simulink model "BD_SER2"  (Simulink 4.1.1)
settings: Solver=ode1  SolverMode=SingleTasking  StartTime=0.0  StopTime=max(cyc_mph(:,1))  FixedStep=1  MaxStep=1  RelTol=1e-3  AbsTol=1e-3
undefined symbols (not defined in the file): air_cp, amb_tmp, cyc_avg_time, cyc_cargo_mass, cyc_elevation_init, cyc_filter_bool, cyc_grade, cyc_mph, enable_stop, ess_cap_scale, ess_coulombic_eff, ess_init_soc, ess_max_ah_cap, ess_max_volts, ess_min_volts, ess_mod_airflow, ess_mod_cp, ess_mod_init_tmp, ess_module_mass, ess_module_num, ess_on, ess_res_scale_coef, ess_res_scale_fun, ess_set_tmp, ess_th_calc, ess_th_res_off, ess_th_res_on, ess_tmp, ess_voc, ex_calc, fc_ct_trq, fc_emis, fc_inertia, fc_map_spd, fc_max_trq, fc_spd_scale, fc_trq_scale, fd_inertia, fd_loss, fd_ratio, gb_dnshift_load, gb_dnshift_spd, gb_gears_num, gb_inertia, gb_num_init, gb_ratio, gb_shift_delay, gb_spd_scale, gb_trq_scale, gb_upshift_load, gb_upshift_spd, gc_inertia, gc_map_spd, gc_map_trq, gc_max_crrnt, gc_max_trq, gc_outpwr_map, gc_overtrq_factor, gc_spd_scale, gc_trq_scale ... (+37)
libraries: lib_wheel2 x12, lib_accessory2 x4, lib_controls2 x3, lib_etc x2, lib_help x2, lib_fuel_converter x2, lib_drive_cycle2 x1, lib_interactive x1, lib_drive_cycle x1, lib_exhaust x1, lib_fuel_converter3 x1
(part 1 of 15)
settings Model: ExecutionOrder=on  LastModifiedBy=mokeefe  ModifiedComment=mokeefe -- Thu Apr 17 14:19:28 2003 -- Version 1.44  SaveTime=off  SaveOutput=off  LimitDataPoints=off  UnconnectedLineMsg=none  RTWOptions="-aEnforceIntegerDowncast=1 -aExtMode=0 -aFoldNonRolledExpr=1 -aForceParamTrailComments=0 -aGenerateComments=1 -aIgnoreCustomStorageClasses=1 -aIncHierarchyInIds=0 -aInlineInvariantSignals=1 -aInlineParameters=0 -aLocalBlockOutputs=1 -aLogVarNameModifier=\"rt_\" -aRTWVerbose=1 -aRollThreshold=5 -aShowEliminatedStatements=1"  RTWTemplateMakefile=grt_vc.tmf  ExtModeTrigMode=oneshot  ExtModeArmWhenConnect=off
settings Model: ModifiedHistory=|
  | mokeefe -- Thu Apr 17 14:19:28 2003 -- Version 1.44
  | 
  | 
  | abrooker -- Tue May 14 11:48:19 2002 -- Version 1.43
  | 
  | 
  | mokeefe -- Thu Apr 18 08:06:50 2002 -- Version 1.42
  | saving the model:
  | o "without the model browser open"
  | o with only top-level screen visible
  | o and with "fit to view" enabled

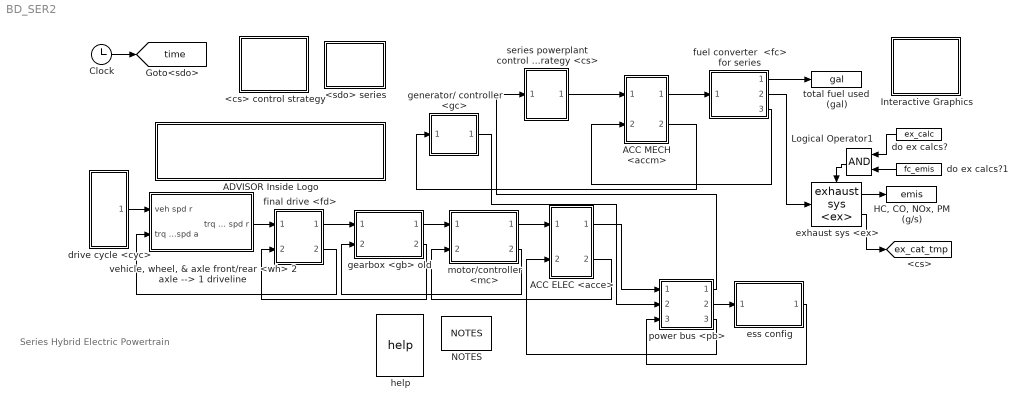
== system BD_SER2 ==
  note: Series Hybrid Electric
      | Powertrain
  <cs> control strategy : Subsystem
      settings: RTWFcnNameOpts=Auto  RTWFileNameOpts=Auto
      mask Display: image(imread('bdi_cs.jpg'))
  <sdo> series : Subsystem
      settings: RTWFcnNameOpts=Auto  RTWFileNameOpts=Auto
      mask Display: image(imread('bdi_sdo.jpg'))
  ACC ELEC <acce> : Subsystem  AncestorBlock=lib_accessory2/ACC ELEC <acce>  mask(Stand-Alone Electrical Accessory Mask){generalName='acce', logPick=Log, initFileName={}, modCell={}, imgFileName='bdi_acc_elec.bmp', DEBUG=OFF}
      mask prompts: generalName "General Name of this Component [char]"; logPick "Log Variables to Workspace?"; initFileName "Initialization File(s) [cell array of char]"; modCell "Modification Cell [2 column cell array of param and val]"; imgFileName "Icon image file name [char--evaluated]"
      mask init:
      | % initialization via m-file script
      | advSACompMaskInit;
      settings: RTWFcnNameOpts=Auto  RTWFileNameOpts=Auto
      mask StyleString: edit,popup(Don't Log|Log),edit,edit,edit,popup(ON|OFF)
      mask Display: image(imread(imgFileName))
  ACC MECH <accm> : Subsystem  AncestorBlock=lib_accessory2/ACC MECH <accm>  mask(Stand-Alone Mechanical Accessory Mask){generalName='accm', logPick=Log, initFileName={}, modCell={}, imgFileName='bdi_acc_pic.bmp', DEBUG=OFF}
      mask prompts: generalName "General Name of this Component [char]"; logPick "Log Variables to Workspace?"; initFileName "Initialization File(s) [cell array of char]"; modCell "Modification Cell [2 column cell array of param and val]"; imgFileName "Icon image file name [char--evaluated]"
      mask init:
      | % initialization via m-file script
      | advSACompMaskInit;
      settings: RTWFcnNameOpts=Auto  RTWFileNameOpts=Auto
      mask StyleString: edit,popup(Don't Log|Log),edit,edit,edit,popup(ON|OFF)
      mask Display: image(imread(imgFileName))
  ADVISOR Inside Logo : Subsystem
      settings: RTWFcnNameOpts=Auto  RTWFileNameOpts=Auto
      mask Display: image(imread('advisorInside.jpg'))
  Clock : Clock
      settings: DisplayTime=off  Decimation=10
  "HC, CO, NOx, PM (g/s)" : ToWorkspace  VariableName=emis  SampleTime=0  SaveFormat=Array
  Interactive Graphics : Subsystem  BlockChoice=off
      settings: AttributesFormatString=%<BlockChoice>  TemplateBlock=lib_interactive/Interactive Graphics  MemberBlocks=off,on  RTWFcnNameOpts=Auto  RTWFileNameOpts=Auto
  Logical Operator1 : Logic  Orientation=left  Operator=AND  Inputs=2
  NOTES : lib_help/NOTES
  do ex calcs? : Constant  Orientation=left  Value=ex_calc
  do ex calcs?1 : Constant  Orientation=left  Value=fc_emis
  drive cycle <cyc> : Subsystem  AncestorBlock=lib_drive_cycle2/drive cycle <cyc>  mask(Stand-Alone Drive Cycle Mask){generalName='cyc', logPick=Log, initFileName={}, modCell={}, imgFileName='bdi_cyc.jpg', DEBUG=OFF, veh_mass=veh_mass}
      mask prompts: generalName "General Name of this Component [char]"; logPick "Log Variables to Workspace?"; initFileName "Initialization File(s) [cell array of char]"; modCell "Modification Cell [2 column cell array of param and val]"; imgFileName "Icon image file name [char--evaluated]"; veh_mass "Vehicle Mass (kg)"
      mask init:
      | % initialization via m-file script
      | advSACompMaskInit;
      settings: RTWFcnNameOpts=Auto  RTWFileNameOpts=Auto
      mask StyleString: edit,popup(Don't Log|Log),edit,edit,edit,popup(ON|OFF),edit
      mask Display: image(imread(imgFileName))
  ess config : Subsystem  BlockChoice=energy storage <ess>
      link override energy storage <ess>/controlTag: GotoTag=essControl
      link override energy storage <ess>/energy storage <ess>/Model/compute current/enhancedToWorkspace2/To Workspace: VariableName=ess_current  SampleTime=-1  SaveFormat=Array
      link override energy storage <ess>/energy storage <ess>/Model/enhancedToWorkspace/To Workspace: VariableName=ess_pwr_out_r  SampleTime=-1  SaveFormat=Array
      link override energy storage <ess>/energy storage <ess>/Model/enhancedToWorkspace1/To Workspace: VariableName=ess_pwr_loss_a  SampleTime=-1  SaveFormat=Array
      link override energy storage <ess>/energy storage <ess>/Model/enhancedToWorkspace2/To Workspace: VariableName=ess_mod_tmp  SampleTime=-1  SaveFormat=Array
      link override energy storage <ess>/energy storage <ess>/Model/enhancedToWorkspace3/To Workspace: VariableName=ess_air_tmp  SampleTime=-1  SaveFormat=Array
      link override energy storage <ess>/energy storage <ess>/Model/enhancedToWorkspace4/To Workspace: VariableName=ess_air_th_pwr  SampleTime=-1  SaveFormat=Array
      link override energy storage <ess>/energy storage <ess>/Model/enhancedToWorkspace5/To Workspace: VariableName=ess_pwr_out_a  SampleTime=-1  SaveFormat=Array
      link override energy storage <ess>/reqOutTag: GotoTag=essReqOut  TagVisibility=global
      link override energy storage <ess>/sensorsTag: GotoTag=essSensors  TagVisibility=global
      settings: AttributesFormatString=%<BlockChoice>  TemplateBlock=lib_energy_storage2/ess config  MemberBlocks="Ultracapacitor  System,energy storage <ess>,energy storage <ess> RC,energy storage <ess> nnet,energy storage <ess> Saber,energy storage <ess> fundamental model,energy storage <ess> optima fundamental model"  RTWFcnNameOpts=Auto  RTWFileNameOpts=Auto
  exhaust sys <ex> : lib_exhaust/exhaust sys <ex>
  final drive <fd> : Subsystem  AncestorBlock=lib_transmission2/final drive <fd>  mask(Stand-Alone Final Drive Mask){generalName='fd', logPick=Log, initFileName={}, modCell={}, imgFileName='bdi_fd.jpg', DEBUG=OFF}
      mask prompts: generalName "General Name of this Component [char]"; logPick "Log Variables to Workspace?"; initFileName "Initialization File(s) [cell array of char]"; modCell "Modification Cell [2 column cell array of param and val]"; imgFileName "Icon image file name [char--evaluated]"
      mask init:
      | % initialization via m-file script
      | advSACompMaskInit;
      settings: RTWFcnNameOpts=Auto  RTWFileNameOpts=Auto
      mask StyleString: edit,popup(Don't Log|Log),edit,edit,edit,popup(ON|OFF)
      mask Display: image(imread(imgFileName))
  fuel converter  <fc> for series : Subsystem  AncestorBlock=|  mask(Stand-Alone IC ENGINE Mask (Series Hybrid)){generalName='fc', logPick=Log, initFileName={}, modCell={}, imgFileName='bdi_fc.jpg', DEBUG=OFF}
      | lib_fuel_converter3/fuel
      | converter
      |  <fc> for series
      mask prompts: generalName "General Name of this Component [char]"; logPick "Log Variables to Workspace?"; initFileName "Initialization File(s) [cell array of char]"; modCell "Modification Cell [2 column cell array of param and val]"; imgFileName "Icon image file name [char--evaluated]"
      mask init:
      | % initialization via m-file script
      | advSACompMaskInit;
      settings: RTWFcnNameOpts=Auto  RTWFileNameOpts=Auto
      mask StyleString: edit,popup(Don't Log|Log),edit,edit,edit,popup(ON|OFF)
      mask Display: image(imread(imgFileName))
  gearbox <gb> old : Subsystem  AncestorBlock=lib_transmission2/gearbox <gb> old  mask(Stand-Alone Gearbox Mask){generalName='gb', logPick=Log, initFileName={}, modCell={}, imgFileName='bdi_gb.jpg', DEBUG=OFF}
      mask prompts: generalName "General Name of this Component [char]"; logPick "Log Variables to Workspace?"; initFileName "Initialization File(s) [cell array of char]"; modCell "Modification Cell [2 column cell array of param and val]"; imgFileName "Icon image file name [char--evaluated]"
      mask init:
      | % initialization via m-file script
      | advSACompMaskInit;
      settings: RTWFcnNameOpts=Auto  RTWFileNameOpts=Auto
      mask StyleString: edit,popup(Don't Log|Log),edit,edit,edit,popup(ON|OFF)
      mask Display: image(imread(imgFileName))
  generator/ controller <gc> : Subsystem  AncestorBlock=lib_electric_machine2/generator// controller <gc>  mask(Stand-Alone Generator/Controller Mask){generalName='gc', logPick=Log, initFileName={}, modCell={}, imgFileName='bdi_mc.jpg', DEBUG=OFF}
      mask prompts: generalName "General Name of this Component [char]"; logPick "Log Variables to Workspace?"; initFileName "Initialization File(s) [cell array of char]"; modCell "Modification Cell [2 column cell array of param and val]"; imgFileName "Icon image file name [char--evaluated]"
      mask init:
      | % initialization via m-file script
      | advSACompMaskInit;
      settings: RTWFcnNameOpts=Auto  RTWFileNameOpts=Auto
      mask StyleString: edit,popup(Don't Log|Log),edit,edit,edit,popup(ON|OFF)
      mask Display: image(imread(imgFileName))
  help : lib_help/help
  motor/controller <mc> : Subsystem  AncestorBlock=lib_electric_machine2/motor//controller <mc>  mask(Stand-Alone Motor/Controller Mask){generalName='mc', logPick=Log, initFileName={}, modCell={}, imgFileName='bdi_mc.jpg', DEBUG=OFF}
      mask prompts: generalName "General Name of this Component [char]"; logPick "Log Variables to Workspace?"; initFileName "Initialization File(s) [cell array of char]"; modCell "Modification Cell [2 column cell array of param and val]"; imgFileName "Icon image file name [char--evaluated]"
      mask init:
      | % initialization via m-file script
      | advSACompMaskInit;
      settings: RTWFcnNameOpts=Auto  RTWFileNameOpts=Auto
      mask StyleString: edit,popup(Don't Log|Log),edit,edit,edit,popup(ON|OFF)
      mask Display: image(imread(imgFileName))
  power bus <pb> : Subsystem  AncestorBlock=lib_power_bus2/power bus <pb>  mask(Stand-Alone Power Bus Mask){generalName='pb', logPick=Log, initFileName={}, modCell={}, imgFileName='bdi_pb.jpg', DEBUG=OFF}
      mask prompts: generalName "General Name of this Component [char]"; logPick "Log Variables to Workspace?"; initFileName "Initialization File(s) [cell array of char]"; modCell "Modification Cell [2 column cell array of param and val]"; imgFileName "Icon image file name [char--evaluated]"
      mask init:
      | % initialization via m-file script
      | advSACompMaskInit;
      settings: RTWFcnNameOpts=Auto  RTWFileNameOpts=Auto
      mask StyleString: edit,popup(Don't Log|Log),edit,edit,edit,popup(ON|OFF)
      mask Display: image(imread(imgFileName))
  series powerplant control strategy <cs> : Subsystem  AncestorBlock=lib_controls2/series powerplant control strategy <cs>  mask(Stand-Alone Series Powerplant Control Strategy Mask){generalName='cs', logPick=Log, initFileName={}, modCell={}, imgFileName='bdi_hybrid_cntrl.jpg', DEBUG=OFF}
      mask prompts: generalName "General Name of this Component [char]"; logPick "Log Variables to Workspace?"; initFileName "Initialization File(s) [cell array of char]"; modCell "Modification Cell [2 column cell array of param and val]"; imgFileName "Icon image file name [char--evaluated]"
      mask init:
      | % initialization via m-file script
      | advSACompMaskInit;
      settings: RTWFcnNameOpts=Auto  RTWFileNameOpts=Auto
      mask StyleString: edit,popup(Don't Log|Log),edit,edit,edit,popup(ON|OFF)
      mask Display: image(imread(imgFileName))
  total fuel used  (gal) : ToWorkspace  VariableName=gal  SampleTime=0  SaveFormat=Array
  "vehicle, wheel, & axle front/rear <wh> 2 axle --> 1 driveline" : Subsystem  AncestorBlock=|  mask(Stand-Alone Vehicle, Wheel, & Axle Mask){generalName='veh', generalName01='wh', logPick=Log, initFileName={}, modCell={}, imgFileName='bdi_wh&veh.jpg', DEBUG=OFF}
      | lib_wheel2/vehicle, wheel, & axle
      | front//rear <wh>
      | 2 axle --> 1 driveline
      mask prompts: generalName "General Name of Vehicle Component [char]"; generalName01 "General Name of Wheel Component [char]"; logPick "Log Variables to Workspace?"; initFileName "Initialization File(s) for VEH and WH [cell array of char]"; modCell "Modification Cell [2 column cell array of param and val]"; imgFileName "Icon image file name [char--evaluated]"
      mask init:
      | % initialization via m-file script
      | advSACompMaskInit;
      settings: RTWFcnNameOpts=Auto  RTWFileNameOpts=Auto
      mask StyleString: edit,edit,popup(Don't Log|Log),edit,edit,edit,popup(ON|OFF)
      mask Display: image(imread(imgFileName))
  tag scope: ex_cat_tmp=global, time=global
  wires:
  gearbox <gb> old/1("torque and speed req'd at input side of gearbox (Nm), (rad/s)") -> motor/controller <mc>/1(trq and spd out requested)
  final drive <fd>/2("torque and speed avail. at output side of final drive (Nm), (rad/s)") -> "vehicle, wheel, & axle front/rear <wh> 2 axle --> 1 driveline"/2(trq & spd a)
  "vehicle, wheel, & axle front/rear <wh> 2 axle --> 1 driveline"/1(trq & spd r) -> final drive <fd>/1("torque and speed req'd at output side of final drive (Nm), (rad/s)")
  gearbox <gb> old/2("torque and speed avail. at output side of gearbox (Nm), (rad/s)") -> final drive <fd>/2("torque and speed avail. at input side of final drive (Nm), (rad/s)")
  final drive <fd>/1("torque and speed req'd at input side of final drive (Nm), (rad/s)") -> gearbox <gb> old/1("torque and speed req'd at output side of gearbox (Nm), (rad/s)")
  drive cycle <cyc>/1(req'd vehicle speed (m/s)) -> "vehicle, wheel, & axle front/rear <wh> 2 axle --> 1 driveline"/1(veh spd r)
  Clock/1 -> [time]
  fuel converter  <fc> for series/2(EO emis info) -> exhaust sys <ex>/1
  fuel converter  <fc> for series/1(fuel use) -> total fuel used  (gal)/1
  Logical Operator1/1 -> exhaust sys <ex>/Enable
  do ex calcs?/1 -> Logical Operator1/1
  exhaust sys <ex>/1 -> "HC, CO, NOx, PM (g/s)"/1
  do ex calcs?1/1 -> Logical Operator1/2
  generator/ controller <gc>/1(generator output power (W)) -> power bus <pb>/2(power available from source one (W))
  ess config/1(power available to bus (W)) -> power bus <pb>/3(power available from source two (W))
  power bus <pb>/2(power req'd from source two (W)) -> ess config/1(power req'd into bus (W))
  motor/controller <mc>/2("trq and spd out achieved ") -> gearbox <gb> old/2("torque and speed avail. at input side of gearbox (Nm), (rad/s)")
  power bus <pb>/1(power req'd from source one (W)) -> series powerplant control strategy <cs>/1(power req'd by bus (W))
  exhaust sys <ex>/2 -> [ex_cat_tmp]
  series powerplant control strategy <cs>/1("engine torque and speed (Nm), (rad/s)") -> ACC MECH <accm>/1(trq and spd out requested)
  ACC MECH <accm>/1(trq and spd in  requested) -> fuel converter  <fc> for series/1(torque and speed  req'd at engine  output shaft (Nm))
  fuel converter  <fc> for series/3("torque and speed  avail. to driveline (Nm), (rad/s)") -> ACC MECH <accm>/2(trq and spd in achieved)
  ACC MECH <accm>/2("trq and spd out achieved ") -> generator/ controller <gc>/1("torque and speed supplied to rotor (Nm), (rad/s)")
  motor/controller <mc>/1(electric power in  requested) -> ACC ELEC <acce>/1(elec pwr out r (W))
  ACC ELEC <acce>/1(elec pwr in r (W)) -> power bus <pb>/1(req'd power output (W))
  power bus <pb>/3(output power  available at bus) -> ACC ELEC <acce>/2(elec pwr in a (W))
  ACC ELEC <acce>/2(elec pwr out a (W)) -> motor/controller <mc>/2(electric power in achieved)

== system BD_SER2/<cs> control strategy ==
  Drive Cycle : Subsystem
      settings: RTWFcnNameOpts=Auto  RTWFileNameOpts=Auto
  Electrical Accessories : Subsystem
      settings: RTWFcnNameOpts=Auto  RTWFileNameOpts=Auto
  Gearbox Control manual shift logic for series : Subsystem
      settings: RTWFcnNameOpts=Auto  RTWFileNameOpts=Auto
  Generator : Subsystem
      settings: RTWFcnNameOpts=Auto  RTWFileNameOpts=Auto
  Hybrid Control Strategy : Subsystem
      settings: RTWFcnNameOpts=Auto  RTWFileNameOpts=Auto
      mask Display: image(imread('bdi_hybrid_cntrl.jpg'))
  IC Engine Control Series Hybrid : Subsystem
      settings: RTWFcnNameOpts=Auto  RTWFileNameOpts=Auto
  Mechanical Accessories : Subsystem
      settings: RTWFcnNameOpts=Auto  RTWFileNameOpts=Auto
  Motor Controller : Subsystem
      settings: RTWFcnNameOpts=Auto  RTWFileNameOpts=Auto
  Power Bus : Subsystem
      settings: RTWFcnNameOpts=Auto  RTWFileNameOpts=Auto
  Wheel Control : Subsystem
      settings: RTWFcnNameOpts=Auto  RTWFileNameOpts=Auto

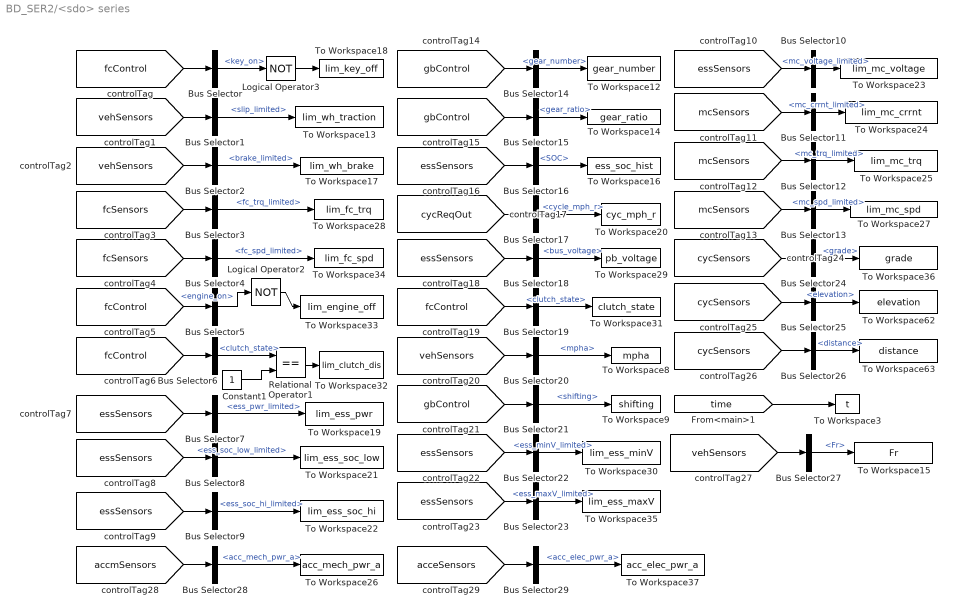
== system BD_SER2/<sdo> series ==
  Bus Selector : BusSelector  OutputSignals=key_on  MuxedOutput=off
  Bus Selector1 : BusSelector  OutputSignals=slip_limited  MuxedOutput=off
  Bus Selector10 : BusSelector  OutputSignals=mc_voltage_limited  MuxedOutput=off
  Bus Selector11 : BusSelector  OutputSignals=mc_crrnt_limited  MuxedOutput=off
  Bus Selector12 : BusSelector  OutputSignals=mc_trq_limited  MuxedOutput=off
  Bus Selector13 : BusSelector  OutputSignals=mc_spd_limited  MuxedOutput=off
  Bus Selector14 : BusSelector  OutputSignals=gear_number  MuxedOutput=off
  Bus Selector15 : BusSelector  OutputSignals=gear_ratio  MuxedOutput=off
  Bus Selector16 : BusSelector  OutputSignals=SOC  MuxedOutput=off
  Bus Selector17 : BusSelector  OutputSignals=cycle_mph_r  MuxedOutput=off
  Bus Selector18 : BusSelector  OutputSignals=bus_voltage  MuxedOutput=off
  Bus Selector19 : BusSelector  OutputSignals=clutch_state  MuxedOutput=off
  Bus Selector2 : BusSelector  OutputSignals=brake_limited  MuxedOutput=off
  Bus Selector20 : BusSelector  OutputSignals=mpha  MuxedOutput=off
  Bus Selector21 : BusSelector  OutputSignals=shifting  MuxedOutput=off
  Bus Selector22 : BusSelector  OutputSignals=ess_minV_limited  MuxedOutput=off
  Bus Selector23 : BusSelector  OutputSignals=ess_maxV_limited  MuxedOutput=off
  Bus Selector24 : BusSelector  OutputSignals=grade  MuxedOutput=off
  Bus Selector25 : BusSelector  OutputSignals=elevation  MuxedOutput=off
  Bus Selector26 : BusSelector  OutputSignals=distance  MuxedOutput=off
  Bus Selector27 : BusSelector  OutputSignals=Fr  MuxedOutput=off
  Bus Selector28 : BusSelector  OutputSignals=acc_mech_pwr_a  MuxedOutput=off
  Bus Selector29 : BusSelector  OutputSignals=acc_elec_pwr_a  MuxedOutput=off
  Bus Selector3 : BusSelector  OutputSignals=fc_trq_limited  MuxedOutput=off
  Bus Selector4 : BusSelector  OutputSignals=fc_spd_limited  MuxedOutput=off
  Bus Selector5 : BusSelector  OutputSignals=engine_on  MuxedOutput=off
  Bus Selector6 : BusSelector  OutputSignals=clutch_state  MuxedOutput=off
  Bus Selector7 : BusSelector  OutputSignals=ess_pwr_limited  MuxedOutput=off
  Bus Selector8 : BusSelector  OutputSignals=ess_soc_low_limited  MuxedOutput=off
  Bus Selector9 : BusSelector  OutputSignals=ess_soc_hi_limited  MuxedOutput=off
  Constant1 : Constant  Value=1
  Logical Operator2 : Logic  Operator=NOT  Inputs=1
  Logical Operator3 : Logic  Operator=NOT  Inputs=1
  Relational Operator1 : RelationalOperator  Operator===
  To Workspace12 : ToWorkspace  VariableName=gear_number  SampleTime=-1  SaveFormat=Array
  To Workspace13 : ToWorkspace  VariableName=lim_wh_traction  SampleTime=-1  SaveFormat=Array
  To Workspace14 : ToWorkspace  VariableName=gear_ratio  SampleTime=-1  SaveFormat=Array
  To Workspace15 : ToWorkspace  VariableName=Fr  SampleTime=-1  SaveFormat=Array
  To Workspace16 : ToWorkspace  VariableName=ess_soc_hist  SampleTime=-1  SaveFormat=Array
  To Workspace17 : ToWorkspace  VariableName=lim_wh_brake  SampleTime=-1  SaveFormat=Array
  To Workspace18 : ToWorkspace  VariableName=lim_key_off  SampleTime=-1  SaveFormat=Array
  To Workspace19 : ToWorkspace  VariableName=lim_ess_pwr  SampleTime=-1  SaveFormat=Array
  To Workspace20 : ToWorkspace  VariableName=cyc_mph_r  SampleTime=-1  SaveFormat=Array
  To Workspace21 : ToWorkspace  VariableName=lim_ess_soc_low  SampleTime=-1  SaveFormat=Array
  To Workspace22 : ToWorkspace  VariableName=lim_ess_soc_hi  SampleTime=-1  SaveFormat=Array
  To Workspace23 : ToWorkspace  VariableName=lim_mc_voltage  SampleTime=-1  SaveFormat=Array
  To Workspace24 : ToWorkspace  VariableName=lim_mc_crrnt  SampleTime=-1  SaveFormat=Array
  To Workspace25 : ToWorkspace  VariableName=lim_mc_trq  SampleTime=-1  SaveFormat=Array
  To Workspace26 : ToWorkspace  VariableName=acc_mech_pwr_a  SampleTime=-1  SaveFormat=Array
  To Workspace27 : ToWorkspace  VariableName=lim_mc_spd  SampleTime=-1  SaveFormat=Array
  To Workspace28 : ToWorkspace  VariableName=lim_fc_trq  SampleTime=-1  SaveFormat=Array
  To Workspace29 : ToWorkspace  VariableName=pb_voltage  SampleTime=-1  SaveFormat=Array
  To Workspace3 : ToWorkspace  VariableName=t  SampleTime=0  SaveFormat=Array
  To Workspace30 : ToWorkspace  VariableName=lim_ess_minV  SampleTime=-1  SaveFormat=Array
  To Workspace31 : ToWorkspace  VariableName=clutch_state  SampleTime=-1  SaveFormat=Array
  To Workspace32 : ToWorkspace  VariableName=lim_clutch_dis  SampleTime=-1  SaveFormat=Array
  To Workspace33 : ToWorkspace  VariableName=lim_engine_off  SampleTime=-1  SaveFormat=Array
  To Workspace34 : ToWorkspace  VariableName=lim_fc_spd  SampleTime=-1  SaveFormat=Array
  To Workspace35 : ToWorkspace  VariableName=lim_ess_maxV  SampleTime=-1  SaveFormat=Array
  To Workspace36 : ToWorkspace  VariableName=grade  SampleTime=-1  SaveFormat=Array
  To Workspace37 : ToWorkspace  VariableName=acc_elec_pwr_a  SampleTime=-1  SaveFormat=Array
  To Workspace62 : ToWorkspace  VariableName=elevation  SampleTime=-1  SaveFormat=Array
  To Workspace63 : ToWorkspace  VariableName=distance  SampleTime=-1  SaveFormat=Array
  To Workspace8 : ToWorkspace  VariableName=mpha  SampleTime=-1  SaveFormat=Array
  To Workspace9 : ToWorkspace  VariableName=shifting  SampleTime=-1  SaveFormat=Array
  wires:
  [time] -> To Workspace3/1
  Logical Operator2/1 -> To Workspace33/1
  Bus Selector1/1 -> To Workspace13/1  "<slip_limited>"
  Logical Operator3/1 -> To Workspace18/1
  [fcControl] -> Bus Selector/1
  Bus Selector/1 -> Logical Operator3/1  "<key_on>"
  [vehSensors] -> Bus Selector1/1
  Bus Selector2/1 -> To Workspace17/1  "<brake_limited>"
  [vehSensors] -> Bus Selector2/1
  [fcSensors] -> Bus Selector3/1
  Bus Selector3/1 -> To Workspace28/1  "<fc_trq_limited>"
  [fcSensors] -> Bus Selector4/1
  Bus Selector4/1 -> To Workspace34/1  "<fc_spd_limited>"
  [fcControl] -> Bus Selector5/1
  Bus Selector5/1 -> Logical Operator2/1  "<engine_on>"
  [fcControl] -> Bus Selector6/1
  Relational Operator1/1 -> To Workspace32/1
  Constant1/1 -> Relational Operator1/2
  Bus Selector6/1 -> Relational Operator1/1  "<clutch_state>"
  [essSensors] -> Bus Selector7/1
  Bus Selector7/1 -> To Workspace19/1  "<ess_pwr_limited>"
  [essSensors] -> Bus Selector8/1
  Bus Selector8/1 -> To Workspace21/1  "<ess_soc_low_limited>"
  [essSensors] -> Bus Selector9/1
  Bus Selector9/1 -> To Workspace22/1  "<ess_soc_hi_limited>"
  [essSensors] -> Bus Selector10/1
  Bus Selector10/1 -> To Workspace23/1  "<mc_voltage_limited>"
  [mcSensors] -> Bus Selector11/1
  Bus Selector11/1 -> To Workspace24/1  "<mc_crrnt_limited>"
  [mcSensors] -> Bus Selector12/1
  Bus Selector12/1 -> To Workspace25/1  "<mc_trq_limited>"
  [mcSensors] -> Bus Selector13/1
  Bus Selector13/1 -> To Workspace27/1  "<mc_spd_limited>"
  [gbControl] -> Bus Selector14/1
  Bus Selector14/1 -> To Workspace12/1  "<gear_number>"
  [gbControl] -> Bus Selector15/1
  Bus Selector15/1 -> To Workspace14/1  "<gear_ratio>"
  [essSensors] -> Bus Selector16/1
  Bus Selector16/1 -> To Workspace16/1  "<SOC>"
  [cycReqOut] -> Bus Selector17/1
  Bus Selector17/1 -> To Workspace20/1  "<cycle_mph_r>"
  [essSensors] -> Bus Selector18/1
  Bus Selector18/1 -> To Workspace29/1  "<bus_voltage>"
  [fcControl] -> Bus Selector19/1
  Bus Selector19/1 -> To Workspace31/1  "<clutch_state>"
  [vehSensors] -> Bus Selector20/1
  Bus Selector20/1 -> To Workspace8/1  "<mpha>"
  [gbControl] -> Bus Selector21/1
  Bus Selector21/1 -> To Workspace9/1  "<shifting>"
  [essSensors] -> Bus Selector22/1
  Bus Selector22/1 -> To Workspace30/1  "<ess_minV_limited>"
  [essSensors] -> Bus Selector23/1
  Bus Selector23/1 -> To Workspace35/1  "<ess_maxV_limited>"
  [cycSensors] -> Bus Selector24/1
  Bus Selector24/1 -> To Workspace36/1  "<grade>"
  [cycSensors] -> Bus Selector25/1
  Bus Selector25/1 -> To Workspace62/1  "<elevation>"
  [cycSensors] -> Bus Selector26/1
  Bus Selector26/1 -> To Workspace63/1  "<distance>"
  [vehSensors] -> Bus Selector27/1
  Bus Selector27/1 -> To Workspace15/1  "<Fr>"
  [accmSensors] -> Bus Selector28/1
  Bus Selector28/1 -> To Workspace26/1  "<acc_mech_pwr_a>"
  [acceSensors] -> Bus Selector29/1
  Bus Selector29/1 -> To Workspace37/1  "<acc_elec_pwr_a>"

== system BD_SER2/ACC ELEC <acce> ==
  note: ELECTRICAL ACCESSORY
      | Interface
  elec pwr out r (W) : Inport  Port=1  LatchInput=off
  elec pwr in a (W) : Inport  Port=2  LatchInput=off
  ACC ELEC model and interface : Subsystem
      settings: RTWFcnNameOpts=Auto  RTWFileNameOpts=Auto
      mask Display: image(imread('bdi_acc_elec.bmp'))
  elec pwr in r (W) : Outport  Port=1
  elec pwr out a (W) : Outport  Port=2
  tag scope: acceReqOut=global, acceSensors=global
  wires:
  ACC ELEC model and interface/4(sensors) -> [acceSensors]
  ACC ELEC model and interface/3("achieved electrical Power, out to the driveline (W)") -> elec pwr out a (W)/1
  ACC ELEC model and interface/2("requested electrical Power, in from the power source (W)") -> elec pwr in r (W)/1
  ACC ELEC model and interface/1(requested out) -> [acceReqOut]
  elec pwr in a (W)/1 -> ACC ELEC model and interface/2(achieved power in from power source (W))
  elec pwr out r (W)/1 -> ACC ELEC model and interface/1("requested electrical Power, out to the driveline (W)")
  [acceControl] -> ACC ELEC model and interface/3(control)

== system BD_SER2/ACC MECH <accm> ==
  note: MECHANICAL ACCESSORY
      | Interface
  trq and spd out requested : Inport  Port=1  LatchInput=off
  trq and spd in achieved : Inport  Port=2  LatchInput=off
  mechanical accessory model and interface : Subsystem  AncestorBlock=lib_accessory2/ACC MECH <accm>/mechanical accessory model and interface
      settings: RTWFcnNameOpts=Auto  RTWFileNameOpts=Auto
  trq and spd in  requested : Outport  Port=1
  "trq and spd out achieved " : Outport  Port=2
  tag scope: accmReqOut=global, accmSensors=global
  wires:
  mechanical accessory model and interface/4(sensors) -> [accmSensors]
  [accmControl] -> mechanical accessory model and interface/3(control)
  mechanical accessory model and interface/1(Out Request) -> [accmReqOut]
  mechanical accessory model and interface/2(T,w in request) -> trq and spd in  requested/1
  trq and spd out requested/1 -> mechanical accessory model and interface/1("T, w out requested")
  trq and spd in achieved/1 -> mechanical accessory model and interface/2("T, w in achieved")
  mechanical accessory model and interface/3("T, w out achieved") -> "trq and spd out achieved "/1

== system BD_SER2/ADVISOR Inside Logo ==

== system BD_SER2/Interactive Graphics ==
  off : lib_interactive/off  Tag=Altia_off  Orientation=up

== system BD_SER2/drive cycle <cyc> ==
  note: DRIVE CYCLE
  drive cycle model and interface : Subsystem
      settings: RTWFcnNameOpts=Auto  RTWFileNameOpts=Auto
  req'd vehicle speed (m/s) : Outport  Port=1  InitialOutput=0
  tag scope: cycReqOut=global, cycSensors=global
  wires:
  drive cycle model and interface/3(sensors) -> [cycSensors]
  drive cycle model and interface/1(req'd lookups) -> [cycReqOut]
  [cycControl] -> drive cycle model and interface/1(control)
  drive cycle model and interface/2(req'd vehicle speed (m/s)) -> req'd vehicle speed (m/s)/1

== system BD_SER2/ess config ==
  power req'd into bus (W) : Inport  Port=1  LatchInput=off
  energy storage <ess> : Subsystem  AncestorBlock=lib_energy_storage2/energy storage <ess>  mask(Stand-Alone Energy Storage System Mask){generalName='ess', logPick=Log Variable, initFileName={}, modCell={}, imgFileName='bdi_ess.jpg', DEBUG=OFF}
      mask prompts: generalName "General Name of this Component [char]"; logPick "Log Variables to Workspace?"; initFileName "Initialization File(s) [cell array of char]"; modCell "Modification Cell [2 column cell array of param and val]"; imgFileName "Icon image file name [char--evaluated]"
      mask init:
      | % initialization via m-file script
      | advSACompMaskInit;
      settings: RTWFcnNameOpts=Auto  RTWFileNameOpts=Auto
      mask StyleString: edit,popup(Don't Log|Log Variable),edit,edit,edit,popup(ON|OFF)
      mask Display: image(imread(imgFileName))
  power available to bus (W) : Outport  Port=1
  wires:
  power req'd into bus (W)/1 -> energy storage <ess>/1(power req'd into bus (W))
  energy storage <ess>/1(power available to bus (W)) -> power available to bus (W)/1

== system BD_SER2/final drive <fd> ==
  "torque and speed req'd at output side of final drive (Nm), (rad/s)" : Inport  Port=1  LatchInput=off
  "torque and speed avail. at input side of final drive (Nm), (rad/s)" : Inport  Port=2  LatchInput=off
  Block NOTES : Subsystem
      settings: RTWFcnNameOpts=Auto  RTWFileNameOpts=Auto
      mask Display: disp('Block\nNOTES')
  help : Subsystem
      settings: OpenFcn=web(['file:\\\' which('wheel_axle.htm')]);  RTWFcnNameOpts=Auto  RTWFileNameOpts=Auto
      mask Display: image(imread('doc_man.jpg'))
  model&interface : Subsystem
      settings: RTWFcnNameOpts=Auto  RTWFileNameOpts=Auto
  "torque and speed req'd at input side of final drive (Nm), (rad/s)" : Outport  Port=1  InitialOutput=0
  "torque and speed avail. at output side of final drive (Nm), (rad/s)" : Outport  Port=2  InitialOutput=0
  tag scope: fdReqOut=global, fdSensors=global
  wires:
  model&interface/3(T & w output achieved) -> "torque and speed avail. at output side of final drive (Nm), (rad/s)"/1
  model&interface/2(T & w input request) -> "torque and speed req'd at input side of final drive (Nm), (rad/s)"/1
  "torque and speed avail. at input side of final drive (Nm), (rad/s)"/1 -> model&interface/2(T & w input achieved)
  "torque and speed req'd at output side of final drive (Nm), (rad/s)"/1 -> model&interface/1(T & w output request)
  model&interface/4(sensors) -> [fdSensors]
  [fdControl] -> model&interface/3(control)
  model&interface/1(out request) -> [fdReqOut]

== system BD_SER2/fuel converter  <fc> for series ==
  note: Internal Combustion Engine
      | for Series Powertrain
  torque and speed  req'd at engine  output shaft (Nm) : Inport  Port=1  LatchInput=off
  Model & Interface : Subsystem
      settings: RTWFcnNameOpts=Auto  RTWFileNameOpts=Auto
  fuel use : Outport  Port=1  InitialOutput=0
  EO emis info : Outport  Port=2  InitialOutput=0
  "torque and speed  avail. to driveline (Nm), (rad/s)" : Outport  Port=3  InitialOutput=0
  tag scope: fcReqOut=global, fcSensors=global
  wires:
  Model & Interface/5(sensors) -> [fcSensors]
  Model & Interface/1(req'd out) -> [fcReqOut]
  [fcControl] -> Model & Interface/2(control)
  Model & Interface/4("torque and speed  avail. to driveline (Nm), (rad/s)") -> "torque and speed  avail. to driveline (Nm), (rad/s)"/1
  Model & Interface/3(EO emis info) -> EO emis info/1
  torque and speed  req'd at engine  output shaft (Nm)/1 -> Model & Interface/1(torque and speed  req'd at engine  output shaft (Nm))
  Model & Interface/2(fuel use) -> fuel use/1

== system BD_SER2/gearbox <gb> old ==
  note: Gearbox
  "torque and speed req'd at output side of gearbox (Nm), (rad/s)" : Inport  Port=1  LatchInput=off
  "torque and speed avail. at input side of gearbox (Nm), (rad/s)" : Inport  Port=2  LatchInput=off
  Block NOTES : Subsystem
      settings: RTWFcnNameOpts=Auto  RTWFileNameOpts=Auto
      mask Display: disp('Block\nNOTES')
  gearbox model & interface : Subsystem
      settings: RTWFcnNameOpts=Auto  RTWFileNameOpts=Auto
  help : Subsystem
      settings: OpenFcn=web(['file:\\\' which('gearbox.htm')]);  RTWFcnNameOpts=Auto  RTWFileNameOpts=Auto
      mask Display: image(imread('doc_man.jpg'))
  "torque and speed req'd at input side of gearbox (Nm), (rad/s)" : Outport  Port=1  InitialOutput=0
  "torque and speed avail. at output side of gearbox (Nm), (rad/s)" : Outport  Port=2  InitialOutput=0
  tag scope: gbReqOut=global, gbSensors=global
  wires:
  gearbox model & interface/4(sensors) -> [gbSensors]
  [gbControl] -> gearbox model & interface/3(controls)
  gearbox model & interface/3(trq and spd output achieved) -> "torque and speed avail. at output side of gearbox (Nm), (rad/s)"/1
  "torque and speed avail. at input side of gearbox (Nm), (rad/s)"/1 -> gearbox model & interface/2(trq and spd input achieved)
  "torque and speed req'd at output side of gearbox (Nm), (rad/s)"/1 -> gearbox model & interface/1(trq and spd output request)
  gearbox model & interface/2(trq and spd input request) -> "torque and speed req'd at input side of gearbox (Nm), (rad/s)"/1
  gearbox model & interface/1(requested output) -> [gbReqOut]

== system BD_SER2/generator/ controller <gc> ==
  note: Generator/ CONTROLLER
      | Interface
  "torque and speed supplied to rotor (Nm), (rad/s)" : Inport  Port=1  LatchInput=off
  GC Model : Subsystem
      settings: RTWFcnNameOpts=Auto  RTWFileNameOpts=Auto
  generator output power (W) : Outport  Port=1  InitialOutput=0
  tag scope: gcReqOut=global, gcSensors=global
  wires:
  GC Model/3(Sensors) -> [gcSensors]
  GC Model/2(generator output power (W)) -> generator output power (W)/1
  GC Model/1(requestedOut) -> [gcReqOut]
  [gcControl] -> GC Model/2(Control)
  "torque and speed supplied to rotor (Nm), (rad/s)"/1 -> GC Model/1("torque and speed supplied to rotor (Nm), (rad/s)")

== system BD_SER2/motor/controller <mc> ==
  note: MOTOR/ CONTROLLER
      | Interface
  trq and spd out requested : Inport  Port=1  LatchInput=off
  electric power in achieved : Inport  Port=2  LatchInput=off
  motor model & interface : Subsystem
      settings: RTWFcnNameOpts=Auto  RTWFileNameOpts=Auto
  electric power in  requested : Outport  Port=1
  "trq and spd out achieved " : Outport  Port=2
  tag scope: mcReqOut=global, mcSensors=global
  wires:
  motor model & interface/3("trq and spd out achieved ") -> "trq and spd out achieved "/1
  electric power in achieved/1 -> motor model & interface/2(electric power in achieved)
  trq and spd out requested/1 -> motor model & interface/1(trq and spd out requested)
  motor model & interface/2(electric power in  requested) -> electric power in  requested/1
  motor model & interface/1(Out Request) -> [mcReqOut]
  [mcControl] -> motor model & interface/3(control)
  motor model & interface/4(sensors) -> [mcSensors]

== system BD_SER2/power bus <pb> ==
  note: Power Bus (PB)
  req'd power output (W) : Inport  Port=1  LatchInput=off
  power available from source one (W) : Inport  Port=2  LatchInput=off
  power available from source two (W) : Inport  Port=3  LatchInput=off
  Block NOTES : Subsystem
      settings: RTWFcnNameOpts=Auto  RTWFileNameOpts=Auto
      mask Display: disp('Block\nNOTES')
  help : Subsystem
      settings: OpenFcn=web(['file:\\\' which('fuel_converter.htm')]);  RTWFcnNameOpts=Auto  RTWFileNameOpts=Auto
      mask Display: image(imread('doc_man.jpg'))
  power bus : Subsystem
      settings: RTWFcnNameOpts=Auto  RTWFileNameOpts=Auto
  power req'd from source one (W) : Outport  Port=1
  power req'd from source two (W) : Outport  Port=2
  output power  available at bus : Outport  Port=3
  tag scope: pbReqOut=global, pbSensors=global
  wires:
  power bus/5(sensors) -> [pbSensors]
  power bus/4(power out available) -> output power  available at bus/1
  power bus/3(power in req from  source two) -> power req'd from source two (W)/1
  power bus/2(power in req from  source one) -> power req'd from source one (W)/1
  power bus/1(required out) -> [pbReqOut]
  [pbControl] -> power bus/4(control)
  power available from source two (W)/1 -> power bus/3(power available from source two)
  power available from source one (W)/1 -> power bus/2(power available from source one)
  req'd power output (W)/1 -> power bus/1(power out req)

== system BD_SER2/series powerplant control strategy <cs> ==
  note: Series Powerplant Control Strategy
  power req'd by bus (W) : Inport  Port=1  LatchInput=off
  Model and Interface : lib_controls2/series powerplant control strategy <cs>/Model and Interface
      settings: RTWFcnNameOpts=Auto  RTWFileNameOpts=Auto
  power follower : lib_controls2/series powerplant control strategy <cs>/power follower
  thermostat : lib_controls2/series powerplant control strategy <cs>/thermostat
  "engine torque and speed (Nm), (rad/s)" : Outport  Port=1  InitialOutput=0
  tag scope: csReqOut=global, csSensors=global
  wires:
  Model and Interface/2 -> "engine torque and speed (Nm), (rad/s)"/1
  power req'd by bus (W)/1 -> Model and Interface/1
  Model and Interface/1 -> [csReqOut]
  [csControl] -> Model and Interface/2
  Model and Interface/3 -> [csSensors]

== system BD_SER2/vehicle, wheel, & axle front/rear <wh> 2 axle --> 1 driveline ==
  note: Vehicle, Wheel, and Axle
      | 2 axles --> 1 driveline
  veh spd r : Inport  Port=1  LatchInput=off
  trq & spd a : Inport  Port=2  LatchInput=off
  models and interface : Subsystem  AncestorBlock=|
      | lib_wheel2/vehicle, wheel, & axle
      | front//rear <wh>
      | 2 axle --> 1 driveline/models and interface
      settings: RTWFcnNameOpts=Auto  RTWFileNameOpts=Auto
  trq & spd r : Outport  Port=1  InitialOutput=0
  tag scope: vehReqOut=global, vehSensors=global
  wires:
  veh spd r/1 -> models and interface/1(vehicle speed req'd at end of time step (m/s))
  trq & spd a/1 -> models and interface/2("torque and speed available from drivetrain into axles (Nm), (rad/s)")
  [vehControl] -> models and interface/3(control)
  models and interface/1(requested out) -> [vehReqOut]
  models and interface/2(torque and speed req'd from drivetrain into axles (Nm),(rad/s)) -> trq & spd r/1
  models and interface/3(sensors) -> [vehSensors]

== system BD_SER2/<cs> control strategy/Drive Cycle ==
  Bus Creator : BusCreator  Inputs=4
  Bus Selector : BusSelector  OutputSignals=mpha  MuxedOutput=off
  Constant : Constant  Value=0
  drive cycle dummy controller : lib_drive_cycle2/drive cycle controls/drive cycle dummy controller
      settings: RTWFcnNameOpts=Auto  RTWFileNameOpts=Auto
  tag scope: cycControl=global
  wires:
  [vehSensors] -> Bus Selector/1
  Bus Selector/1 -> drive cycle dummy controller/1  "<mpha>"
  Constant/1 -> drive cycle dummy controller/3, drive cycle dummy controller/2, drive cycle dummy controller/4
  drive cycle dummy controller/1 -> Bus Creator/1  "mpha"
  drive cycle dummy controller/2 -> Bus Creator/2  "altia_grade"
  drive cycle dummy controller/3 -> Bus Creator/3  "Altia_Run"
  drive cycle dummy controller/4 -> Bus Creator/4  "altia_cyc_mph_r"
  Bus Creator/1 -> [cycControl]

== system BD_SER2/<cs> control strategy/Electrical Accessories ==
  Bus Creator : BusCreator  Inputs=4
  Bus Selector1 : BusSelector  OutputSignals=F_req  MuxedOutput=off
  Bus Selector2 : BusSelector  OutputSignals=key_on  MuxedOutput=off
  Bus Selector3 : BusSelector  OutputSignals=engine_on  MuxedOutput=off
  Constant : Constant  Value=ess_on*1
  electrical accessory controller : Subsystem
      settings: RTWFcnNameOpts=Auto  RTWFileNameOpts=Auto
  tag scope: acceControl=global
  wires:
  Constant/1 -> electrical accessory controller/1(electrical accessories on?)
  Bus Creator/1 -> [acceControl]
  [fcControl] -> Bus Selector2/1
  Bus Selector2/1 -> electrical accessory controller/3(key_on in)  "<key_on>"
  [fcControl] -> Bus Selector3/1
  Bus Selector3/1 -> electrical accessory controller/4(engine_on in)  "<engine_on>"
  [vehReqOut] -> Bus Selector1/1
  Bus Selector1/1 -> electrical accessory controller/2(F_req in)  "<F_req>"
  electrical accessory controller/1(acc_on) -> Bus Creator/1  "acc_on"
  electrical accessory controller/2(F_req) -> Bus Creator/2  "F_req"
  electrical accessory controller/3(key_on) -> Bus Creator/3  "key_on"
  electrical accessory controller/4(engine_on) -> Bus Creator/4  "engine_on"

== system BD_SER2/<cs> control strategy/Gearbox Control manual shift logic for series ==
  Bus Selector1 : BusSelector  OutputSignals=mpha  MuxedOutput=off
  Bus Selector10 : BusSelector  OutputSignals=eta_gb  MuxedOutput=off
  Bus Selector2 : BusSelector  OutputSignals=cycle_mph_r  MuxedOutput=off
  Bus Selector3 : BusSelector  OutputSignals=veh_spd_a_rec  MuxedOutput=off
  Bus Selector4 : BusSelector  OutputSignals=slip_limited  MuxedOutput=off
  Bus Selector7 : BusSelector  OutputSignals=gb_trq_out_r  MuxedOutput=off
  Bus Selector8 : BusSelector  OutputSignals=gb_spd_out_r  MuxedOutput=off
  Bus Selector9 : BusSelector  OutputSignals=gb_spd_in_a  MuxedOutput=off
  Memory : Memory  X0=0  InheritSampleTime=off
      settings: RTWStateStorageClass=Auto
  Memory1 : Memory  X0=0  InheritSampleTime=off
      settings: RTWStateStorageClass=Auto
  Memory2 : Memory  X0=cyc_mph(1,2)  InheritSampleTime=off
      settings: RTWStateStorageClass=Auto
  Memory3 : Memory  X0=0  InheritSampleTime=off
      settings: RTWStateStorageClass=Auto
  Memory4 : Memory  X0=cyc_mph(1,2)  InheritSampleTime=off
      settings: RTWStateStorageClass=Auto
  Mux1 : Mux  Inputs=3
  manual shift logic for series : Subsystem  TreatAsAtomicUnit=on
      settings: RTWFcnNameOpts=Auto  RTWFileNameOpts=Auto
  tag scope: gbControl=global
  wires:
  Memory4/1 -> manual shift logic for series/6("cyc_mph_r, t=(i-1)")
  Memory3/1 -> manual shift logic for series/7("veh_spd_a_rec, t=(i-1)")
  Memory2/1 -> manual shift logic for series/5("mpha, t=(i-1)")
  Memory1/1 -> manual shift logic for series/2("gb_spd_in_a, t=(i-1)")
  Memory/1 -> manual shift logic for series/1("eta_gb, t=(i-1)")
  [gbReqOut] -> Bus Selector7/1, Bus Selector8/1
  Bus Selector7/1 -> manual shift logic for series/4(T_gb_out)  "<gb_trq_out_r>"
  Bus Selector8/1 -> manual shift logic for series/3(w_gb_out)  "<gb_spd_out_r>"
  Bus Selector9/1 -> Memory1/1  "<gb_spd_in_a>"
  Bus Selector10/1 -> Memory/1  "<eta_gb>"
  [gbSensors] -> Bus Selector9/1, Bus Selector10/1
  Mux1/1 -> [gbControl]
  manual shift logic for series/3(gear number) -> Mux1/3  "gear_number"
  manual shift logic for series/2(shifting) -> Mux1/2  "shifting"
  manual shift logic for series/1(gear ratio) -> Mux1/1  "gear_ratio"
  [vehSensors] -> Bus Selector1/1
  Bus Selector1/1 -> Memory2/1  "<mpha>"
  [cycReqOut] -> Bus Selector2/1
  Bus Selector2/1 -> Memory4/1  "<cycle_mph_r>"
  [vehSensors] -> Bus Selector3/1
  Bus Selector3/1 -> Memory3/1  "<veh_spd_a_rec>"
  [vehReqOut] -> Bus Selector4/1
  Bus Selector4/1 -> manual shift logic for series/8(slip_limited)  "<slip_limited>"

== system BD_SER2/<cs> control strategy/Generator ==
  Bus Creator : BusCreator  Inputs=1
  Bus Selector : BusSelector  OutputSignals=bus_voltage  MuxedOutput=off
  Memory : Memory  X0=ess_module_num*mean(ess_voc(1,:))  InheritSampleTime=off
      settings: RTWStateStorageClass=Auto
  generator controller : Subsystem
      settings: RTWFcnNameOpts=Auto  RTWFileNameOpts=Auto
  tag scope: gcControl=global
  wires:
  generator controller/1(bus voltage previous out) -> Bus Creator/1  "bus_voltage_prev"
  Bus Creator/1 -> [gcControl]
  [essSensors] -> Bus Selector/1
  Bus Selector/1 -> Memory/1  "<bus_voltage>"
  Memory/1 -> generator controller/1(bus voltage previous in)

== system BD_SER2/<cs> control strategy/Hybrid Control Strategy ==
  Bus Creator : BusCreator  Inputs=4
  Bus Selector : BusSelector  OutputSignals=ess_max_pwr  MuxedOutput=off
  Bus Selector1 : BusSelector  OutputSignals=SOC  MuxedOutput=off
  Bus Selector2 : BusSelector  OutputSignals=ess_max_chg_pwr  MuxedOutput=off
  Bus Selector3 : BusSelector  OutputSignals=key_on  MuxedOutput=off
  hybrid controls : Subsystem
      settings: RTWFcnNameOpts=Auto  RTWFileNameOpts=Auto
  tag scope: csControl=global
  wires:
  hybrid controls/1(ess_max_pwr out) -> Bus Creator/1  "ess_max_pwr"
  Bus Creator/1 -> [csControl]
  [essSensors] -> Bus Selector/1
  Bus Selector/1 -> hybrid controls/1(ess_max_pwr)  "<ess_max_pwr>"
  hybrid controls/2(SOC in) -> Bus Creator/2  "SOC"
  hybrid controls/3(ess_max_chg_pwr out) -> Bus Creator/3  "ess_max_chg_pwr"
  hybrid controls/4(key_on out) -> Bus Creator/4  "key_on"
  [essSensors] -> Bus Selector1/1
  Bus Selector1/1 -> hybrid controls/2(SOC)  "<SOC>"
  [essSensors] -> Bus Selector2/1
  Bus Selector2/1 -> hybrid controls/3(ess_max_chg_pwr)  "<ess_max_chg_pwr>"
  [fcControl] -> Bus Selector3/1
  Bus Selector3/1 -> hybrid controls/4(key_on)  "<key_on>"

== system BD_SER2/<cs> control strategy/IC Engine Control Series Hybrid ==
  note: Controls for Fuel Converter:
      | IC Engine for Parallel Hybrid
  Bus Creator : BusCreator  Inputs=5
  Bus Selector1 : BusSelector  OutputSignals=engine_on  MuxedOutput=off
  Bus Selector3 : BusSelector  OutputSignals=acc_mech_trq_a  MuxedOutput=off
  Bus Selector6 : BusSelector  OutputSignals=v_prev  MuxedOutput=off
  Fuel Converter Control : Subsystem
      settings: RTWFcnNameOpts=Auto  RTWFileNameOpts=Auto
  Memory : Memory  X0=0  InheritSampleTime=off
      settings: RTWStateStorageClass=Auto
  tag scope: fcControl=global
  wires:
  [csSensors] -> Bus Selector1/1
  [accmSensors] -> Bus Selector3/1
  [vehSensors] -> Bus Selector6/1
  Bus Creator/1 -> [fcControl]
  Fuel Converter Control/1(clutch state out) -> Bus Creator/1  "clutch_state"
  Fuel Converter Control/2(acc_mech_trq_est out) -> Bus Creator/2  "acc_mech_trq_est"
  Fuel Converter Control/3(engine_on out) -> Bus Creator/3  "engine_on"
  Fuel Converter Control/5(key_on out) -> Bus Creator/4  "key_on"
  Fuel Converter Control/4(v_prev out) -> Bus Creator/5  "v_prev"
  [fcSensors] -> Fuel Converter Control/3(fcSensors)
  Bus Selector6/1 -> Fuel Converter Control/4(v_prev)  "<v_prev>"
  Bus Selector3/1 -> Memory/1  "<acc_mech_trq_a>"
  Bus Selector1/1 -> Fuel Converter Control/1(engine_on in)  "<engine_on>"
  Memory/1 -> Fuel Converter Control/2(acc_mech_trq_est)

== system BD_SER2/<cs> control strategy/Mechanical Accessories ==
  Bus Creator : BusCreator  Inputs=9
  Bus Selector : BusSelector  OutputSignals=fc_spd_est  MuxedOutput=off
  Bus Selector1 : BusSelector  OutputSignals=F_req  MuxedOutput=off
  Bus Selector2 : BusSelector  OutputSignals=key_on  MuxedOutput=off
  Bus Selector3 : BusSelector  OutputSignals=engine_on  MuxedOutput=off
  Constant : Constant  Value=not(ess_on)*1
  Constant1 : Constant  Value=inf
  Constant2 : Constant  Value=vc_idle_spd+eps
  mechanical accessory controller : Subsystem
      settings: RTWFcnNameOpts=Auto  RTWFileNameOpts=Auto
  tag scope: accmControl=global
  wires:
  Constant1/1 -> mechanical accessory controller/2(maximum accessory speed)
  Constant2/1 -> mechanical accessory controller/3(minimum accessory speed)
  Constant/1 -> mechanical accessory controller/4(electrical accessories on?)
  mechanical accessory controller/1(acc_on) -> Bus Creator/1
  mechanical accessory controller/2(acc_mech_spd_r) -> Bus Creator/2
  mechanical accessory controller/3(acc_mech_spd_a) -> Bus Creator/3
  mechanical accessory controller/4(acc_max_spd) -> Bus Creator/4
  mechanical accessory controller/5(acc_min_spd) -> Bus Creator/5
  mechanical accessory controller/6(elec_acc_on_bool) -> Bus Creator/6
  mechanical accessory controller/7(F_req) -> Bus Creator/7
  mechanical accessory controller/8(key_on) -> Bus Creator/8
  mechanical accessory controller/9(engine_on) -> Bus Creator/9
  Bus Creator/1 -> [accmControl]
  [fcControl] -> Bus Selector2/1
  Bus Selector2/1 -> mechanical accessory controller/6(key on?)  "<key_on>"
  [fcControl] -> Bus Selector3/1
  Bus Selector3/1 -> mechanical accessory controller/7(engine on?)  "<engine_on>"
  [fcSensors] -> Bus Selector/1
  Bus Selector/1 -> mechanical accessory controller/1(accessory reference shaft speed)  "<fc_spd_est>"
  [vehReqOut] -> Bus Selector1/1
  Bus Selector1/1 -> mechanical accessory controller/5(Force required for vehicle motion)  "<F_req>"
